simulink model "functions"  (R2017a)
settings: Solver=FixedStepDiscrete  StartTime=0.0  StopTime=10.0  FixedStep=0.1  RelTol=1e-3  EnableMultiTasking=on
libraries: simulink x1
settings Model: Creator=thr  LastModifiedBy=thr
settings SolverCC: AutoInsertRateTranBlk=on
settings DataIOCC: LimitDataPoints=on
settings OptimizationCC: LifeSpan=inf
settings DebuggingCC: AllowSymbolicDim=off  SFUnexpectedBacktrackingDiag=warning  SFNoUnconditionalDefaultTransitionDiag=warning  SFExecutionAtInitializationDiag=none
settings GRTTargetCC: TargetLangStandard=C89/C90 (ANSI)  GeneratePreprocessorConditionals=Disable all
settings ConfigComp: CovMetricSettings=dw  CovHtmlReporting=on  CovSaveCumulativeToWorkspaceVar=on  CovSaveSingleToWorkspaceVar=on  CovShowResultsExplorer=off  CovExternalEMLEnable=off  CovSFcnEnable=off

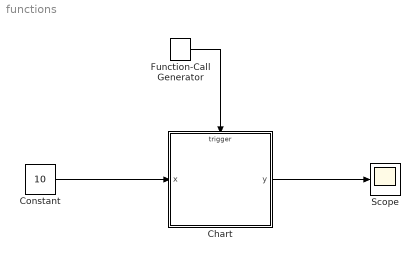
== system functions ==
  Chart : Stateflow chart  TreatAsAtomicUnit=on
  Constant : Constant  Value=10  OutDataTypeStr=int32
  Function-Call Generator : simulink/Ports & Subsystems/Function-Call Generator  sample_time=1  numberOfIterations=1
  Scope : Scope
  wires:
  Function-Call Generator/1 -> Chart/Trigger
  Chart/1(y) -> Scope/1
  Constant/1 -> Chart/1(x)

== stateflow chart functions/Chart ==
  settings: executeAtInitialization=1
  state S1
  state fodo [function]
    (default) -> (junction 6)
    (junction 6) -> (junction 12) [order 1] : [x>9]{y=1}
    (junction 6) -> (junction 14) [order 2] : {y=0}
  state S2
  (default) -> S1
  S1 -> S2 : e{fodo}
  data: y output int32; x input int32
  events: e input FUNCTION_CALL_EVENT
